simulink model "AnalogControl"  (Simulink 8.5)
settings: Solver=ode45  StartTime=0.0  StopTime=10.0  MaxStep=0.1  RelTol=1e-3
undefined symbols (not defined in the file): Ka, Kf, Ki, Kq, Tal, Ts, W1, W2
libraries: simulink x1
settings Model: Creator=The MathWorks Inc.  LastModifiedBy=The MathWorks Inc.  CovSFcnEnable=off
settings DataIOCC: SignalLoggingSaveFormat=Dataset  SaveOutput=off  SaveTime=off  SignalLoggingName=AnalogControl
settings OptimizationCC: InlineParams=on  InitFltsAndDblsToZero=on  SimCompilerOptimization=Off
settings DebuggingCC: SaveWithParameterizedLinksMsg=none  SignalResolutionControl=TryResolveAllWithWarning  SolverPrmCheckMsg=warning  MultiTaskDSMMsg=warning  MultiTaskCondExecSysMsg=none  FcnCallInpInsideContextMsg=UseLocalSettings
settings RTWCC: RTWCompilerOptimization=Off
settings GRTTargetCC: TargetFcnLib=ansi_tfl_tmw.mat

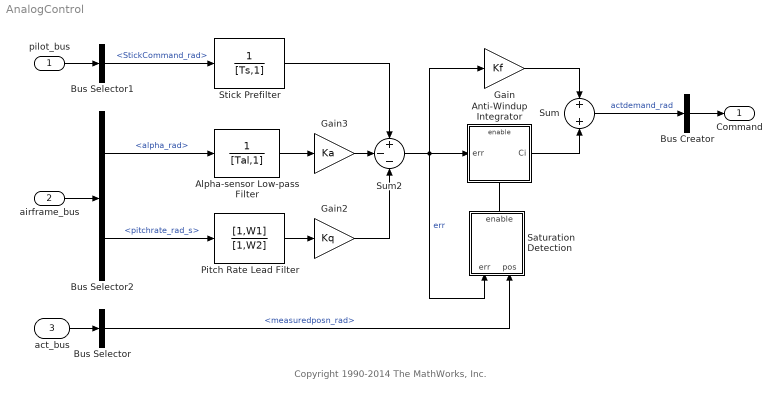
== system AnalogControl ==
  note: Copyright 1990-2014 The MathWorks, Inc.
  pilot_bus : Inport  IOType=none  Commented=off  StatePerturbationForJacobian=1.0e-05  OutDataTypeStr=Bus: PILOT_BUS
  airframe_bus : Inport  IOType=none  Commented=off  StatePerturbationForJacobian=1.0e-05  Port=2  OutDataTypeStr=Bus: AIRFRAME_BUS
  act_bus : Inport  IOType=none  Commented=off  StatePerturbationForJacobian=1.0e-05  Port=3  OutDataTypeStr=Bus: ACT_BUS
  Alpha-sensor Low-pass Filter : TransferFcn  IOType=none  Commented=off  StatePerturbationForJacobian=1.0e-05  Denominator=[Tal,1]
  Anti-Windup Integrator : Subsystem  IOType=none  Commented=off  StatePerturbationForJacobian=1.0e-05  TreatAsAtomicUnit=on
      settings: RTWSystemCode=Inline
  Bus Creator : BusCreator  IOType=none  Commented=off  StatePerturbationForJacobian=1.0e-05  Inputs=1  OutDataTypeStr=Bus: CONTROL_BUS
  Bus Selector : BusSelector  IOType=none  Commented=off  StatePerturbationForJacobian=1.0e-05  OutputSignals=measuredposn_rad
  Bus Selector1 : BusSelector  IOType=none  Commented=off  StatePerturbationForJacobian=1.0e-05  OutputSignals=StickCommand_rad
  Bus Selector2 : BusSelector  IOType=none  Commented=off  StatePerturbationForJacobian=1.0e-05  OutputSignals=alpha_rad,pitchrate_rad_s
  Gain : Gain  IOType=none  Commented=off  StatePerturbationForJacobian=1.0e-05  Gain=Kf  SaturateOnIntegerOverflow=on  OutDataTypeStr=Inherit: Same as input  ParamDataTypeStr=Inherit: Same as input
  Gain2 : Gain  IOType=none  Commented=off  StatePerturbationForJacobian=1.0e-05  Gain=Kq  SaturateOnIntegerOverflow=on  OutDataTypeStr=Inherit: Same as input  ParamDataTypeStr=Inherit: Same as input
  Gain3 : Gain  IOType=none  Commented=off  StatePerturbationForJacobian=1.0e-05  Gain=Ka  SaturateOnIntegerOverflow=on  OutDataTypeStr=Inherit: Same as input  ParamDataTypeStr=Inherit: Same as input
  Pitch Rate Lead Filter : TransferFcn  IOType=none  Commented=off  StatePerturbationForJacobian=1.0e-05  Numerator=[1,W1]  Denominator=[1,W2]
  Saturation Detection : Subsystem  IOType=none  Commented=off  StatePerturbationForJacobian=1.0e-05
  Stick Prefilter : TransferFcn  IOType=none  Commented=off  StatePerturbationForJacobian=1.0e-05  Denominator=[Ts,1]
  Sum : Sum  IOType=none  Commented=off  StatePerturbationForJacobian=1.0e-05  Inputs=2  SaturateOnIntegerOverflow=on  InputSameDT=on  OutDataTypeStr=Inherit: Same as first input
  Sum2 : Sum  IOType=none  Commented=off  StatePerturbationForJacobian=1.0e-05  Inputs=+--  SaturateOnIntegerOverflow=on  InputSameDT=on  OutDataTypeStr=Inherit: Same as first input
  Command : Outport  IOType=none  Commented=off  StatePerturbationForJacobian=1.0e-05  OutDataTypeStr=Bus: CONTROL_BUS
  wires:
  Saturation Detection/1(enable) -> Anti-Windup Integrator/Enable
  Bus Selector/1 -> Saturation Detection/2(pos)  "<measuredposn_rad>"
  Bus Selector2/2 -> Pitch Rate Lead Filter/1  "<pitchrate_rad_s>"
  Bus Selector2/1 -> Alpha-sensor Low-pass Filter/1  "<alpha_rad>"
  Gain/1 -> Sum/1
  Gain3/1 -> Sum2/2
  Pitch Rate Lead Filter/1 -> Gain2/1
  Stick Prefilter/1 -> Sum2/1
  Gain2/1 -> Sum2/3
  Alpha-sensor Low-pass Filter/1 -> Gain3/1
  Bus Selector1/1 -> Stick Prefilter/1  "<StickCommand_rad>"
  Anti-Windup Integrator/1(Ci) -> Sum/2
  Sum2/1 -> Saturation Detection/1(err), Anti-Windup Integrator/1(err), Gain/1  "err"
  pilot_bus/1 -> Bus Selector1/1
  act_bus/1 -> Bus Selector/1
  airframe_bus/1 -> Bus Selector2/1
  Sum/1 -> Bus Creator/1  "actdemand_rad"
  Bus Creator/1 -> Command/1

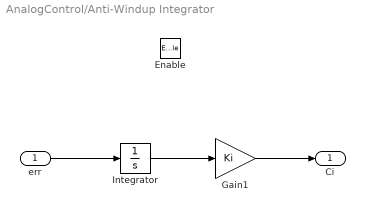
== system AnalogControl/Anti-Windup Integrator ==
  err : Inport  IOType=none  Commented=off  StatePerturbationForJacobian=1.0e-05
  Enable : EnablePort  IOType=none  Commented=off  StatePerturbationForJacobian=1.0e-05
  Gain1 : Gain  IOType=none  Commented=off  StatePerturbationForJacobian=1.0e-05  Gain=Ki  SaturateOnIntegerOverflow=on  OutDataTypeStr=Inherit: Same as input  ParamDataTypeStr=Inherit: Same as input
  Integrator : Integrator  IOType=none  Commented=off  StatePerturbationForJacobian=1.0e-05
  Ci : Outport  IOType=none  Commented=off  StatePerturbationForJacobian=1.0e-05  InitialOutput=0
  wires:
  Gain1/1 -> Ci/1
  Integrator/1 -> Gain1/1
  err/1 -> Integrator/1

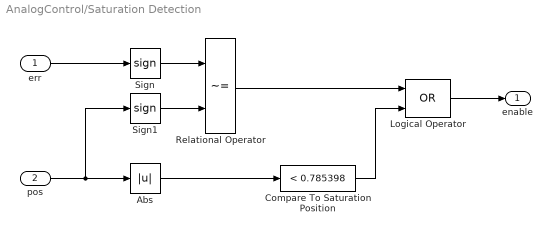
== system AnalogControl/Saturation Detection ==
  err : Inport  IOType=none  Commented=off  StatePerturbationForJacobian=1.0e-05
  pos : Inport  IOType=none  Commented=off  StatePerturbationForJacobian=1.0e-05  Port=2
  Abs : Abs  IOType=none  Commented=off  StatePerturbationForJacobian=1.0e-05  ZeroCross=off
  Compare To Saturation Position : simulink/Logic and Bit Operations/Compare To Constant  IOType=none  Commented=off  StatePerturbationForJacobian=1.0e-05  relop=<  const=0.785398  OutDataTypeStr=boolean  ZeroCross=off
  Logical Operator : Logic  IOType=none  Commented=off  StatePerturbationForJacobian=1.0e-05  Operator=OR  AllPortsSameDT=off  OutDataTypeStr=boolean
  Relational Operator : RelationalOperator  IOType=none  Commented=off  StatePerturbationForJacobian=1.0e-05  Operator=~=  OutDataTypeStr=boolean  ZeroCross=off
  Sign : Signum  IOType=none  Commented=off  StatePerturbationForJacobian=1.0e-05  ZeroCross=off
  Sign1 : Signum  IOType=none  Commented=off  StatePerturbationForJacobian=1.0e-05  ZeroCross=off
  enable : Outport  IOType=none  Commented=off  StatePerturbationForJacobian=1.0e-05
  wires:
  Logical Operator/1 -> enable/1
  err/1 -> Sign/1
  Abs/1 -> Compare To Saturation Position/1
  Sign1/1 -> Relational Operator/2
  Compare To Saturation Position/1 -> Logical Operator/2
  Relational Operator/1 -> Logical Operator/1
  Sign/1 -> Relational Operator/1
  pos/1 -> Abs/1, Sign1/1
